simulink model "FMCW_Target_Emulator_RevA"  (R2021b)
settings: Solver=VariableStepAuto  StartTime=0.0  StopTime=stop_time  RelTol=1e-3
values from neighbouring files (symbols this model uses):
  simulator = Simulator_revB()    [compute_sensed_targets.m]    (also in compute_sensed_values.m)
undefined symbols (not defined in the file or in its folder): emulated_target
libraries: hdlsllib x2, simulink x1
settings Model: SimulationMode=accelerator  Creator=David  LastModifiedBy=David

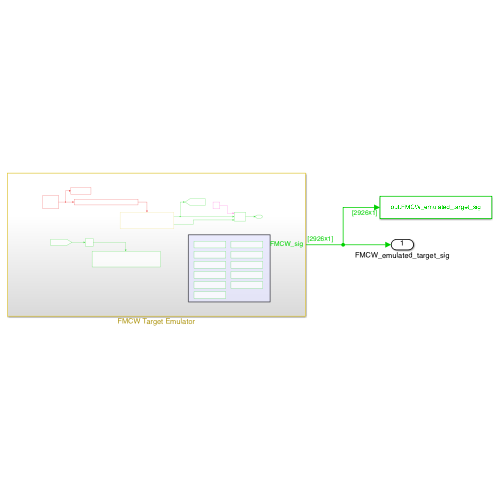
[thumbnail: Simulink's stored preview of the top-level diagram]
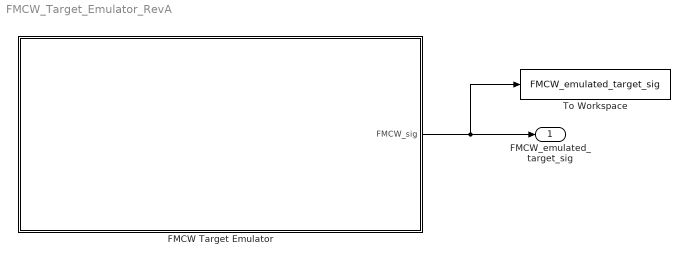
== system FMCW_Target_Emulator_RevA ==
  FMCW Target Emulator : Subsystem
  To Workspace : ToWorkspace  VariableName=FMCW_emulated_target_sig  SampleTime=-1
      settings: MaxDataPoints=2
  FMCW_emulated_target_sig : Outport
  wires:
  FMCW Target Emulator/1(FMCW_sig) -> FMCW_emulated_target_sig/1, To Workspace/1

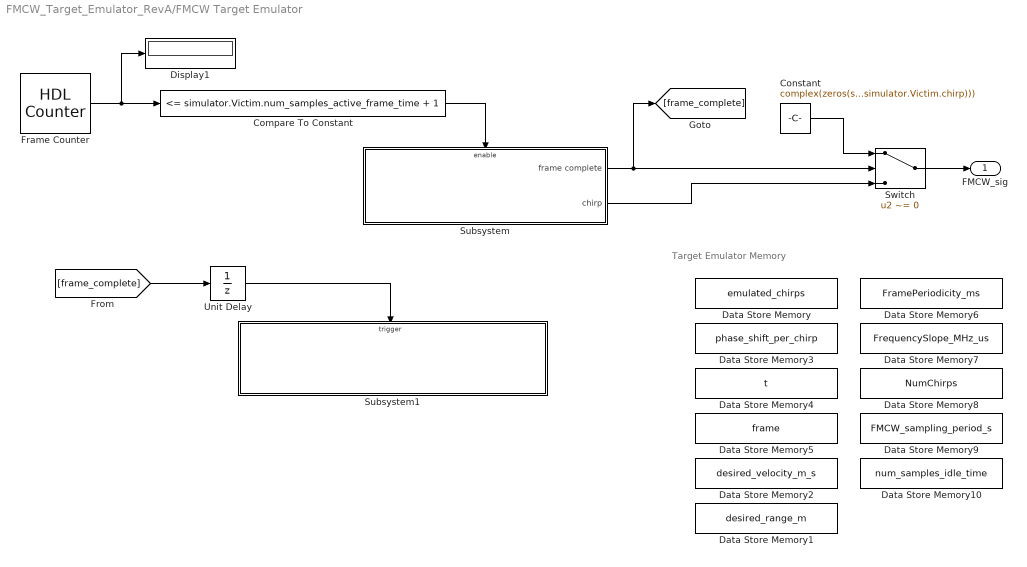
== system FMCW_Target_Emulator_RevA/FMCW Target Emulator ==
  note: Target Emulator Memory
  Compare To Constant : simulink/Logic and Bit Operations/Compare To Constant  relop=<=  const=simulator.Victim.num_samples_active_frame_time + 1  OutDataTypeStr=boolean
  Constant : Constant  Value=complex(zeros(size(simulator.Victim.chirp)))  VectorParams1D=off
  Data Store Memory : DataStoreMemory  DataStoreName=emulated_chirps  ReadBeforeWriteMsg=warning  WriteAfterWriteMsg=warning  WriteAfterReadMsg=warning  InitialValue=emulated_target.emulated_chirps  VectorParams1D=off  ShowAdditionalParam=off  OutDataTypeStr=double  Dimensions=size(emulated_target.emulated_chirps)
      settings: SignalType=complex
  Data Store Memory1 : DataStoreMemory  DataStoreName=desired_range_m  ReadBeforeWriteMsg=warning  WriteAfterWriteMsg=warning  WriteAfterReadMsg=warning  InitialValue=emulated_target.desired_range_m  ShowAdditionalParam=off  OutDataTypeStr=double
  Data Store Memory10 : DataStoreMemory  DataStoreName=num_samples_idle_time  ReadBeforeWriteMsg=warning  WriteAfterWriteMsg=warning  WriteAfterReadMsg=warning  InitialValue=emulated_target.Radar.num_samples_idle_time  ShowAdditionalParam=off  OutDataTypeStr=double
  Data Store Memory2 : DataStoreMemory  DataStoreName=desired_velocity_m_s  ReadBeforeWriteMsg=warning  WriteAfterWriteMsg=warning  WriteAfterReadMsg=warning  InitialValue=emulated_target.desired_velocity_m_s  ShowAdditionalParam=off  OutDataTypeStr=double
  Data Store Memory3 : DataStoreMemory  DataStoreName=phase_shift_per_chirp  ReadBeforeWriteMsg=warning  WriteAfterWriteMsg=warning  WriteAfterReadMsg=warning  InitialValue=emulated_target.phase_shift_per_chirp  ShowAdditionalParam=off  OutDataTypeStr=double
  Data Store Memory4 : DataStoreMemory  DataStoreName=t  ReadBeforeWriteMsg=warning  WriteAfterWriteMsg=warning  WriteAfterReadMsg=warning  InitialValue=emulated_target.t  ShowAdditionalParam=off  OutDataTypeStr=double  Dimensions=size(emulated_target.t)
  Data Store Memory5 : DataStoreMemory  DataStoreName=frame  ReadBeforeWriteMsg=warning  WriteAfterWriteMsg=warning  WriteAfterReadMsg=warning  InitialValue=1  ShowAdditionalParam=off  OutDataTypeStr=double
  Data Store Memory6 : DataStoreMemory  DataStoreName=FramePeriodicity_ms  ReadBeforeWriteMsg=warning  WriteAfterWriteMsg=warning  WriteAfterReadMsg=warning  InitialValue=emulated_target.Radar.FramePeriodicity_ms  ShowAdditionalParam=off  OutDataTypeStr=double
  Data Store Memory7 : DataStoreMemory  DataStoreName=FrequencySlope_MHz_us  ReadBeforeWriteMsg=warning  WriteAfterWriteMsg=warning  WriteAfterReadMsg=warning  InitialValue=emulated_target.Radar.FrequencySlope_MHz_us  ShowAdditionalParam=off  OutDataTypeStr=double
  Data Store Memory8 : DataStoreMemory  DataStoreName=NumChirps  ReadBeforeWriteMsg=warning  WriteAfterWriteMsg=warning  WriteAfterReadMsg=warning  InitialValue=emulated_target.Radar.NumChirps  ShowAdditionalParam=off  OutDataTypeStr=int32
  Data Store Memory9 : DataStoreMemory  DataStoreName=FMCW_sampling_period_s  ReadBeforeWriteMsg=warning  WriteAfterWriteMsg=warning  WriteAfterReadMsg=warning  InitialValue=emulated_target.Radar.FMCW_sampling_period_s  ShowAdditionalParam=off  OutDataTypeStr=double
  Display1 : Display
  Frame Counter : hdlsllib/Sources/HDL Counter  CountType=Count limited  CountInit=1  CountStep=1  CountMax=simulator.Victim.num_samples_per_frame  CountFromType=Initial value  CountFrom=1  CountResetPort=off  CountLoadPort=off  CountEnbPort=off  CountDirPort=off  CountHitOutputPort=off  CountDataType=Unsigned  CountWordLen=32  CountFracLen=0  CountSampTime=1/simulator.Victim.FMCW_sampling_rate_Hz
  Subsystem : Subsystem
  Subsystem1 : Subsystem
  Switch : Switch  Criteria=u2 ~= 0
  Unit Delay : UnitDelay  SampleTime=-1  HasFrameUpgradeWarning=on
  FMCW_sig : Outport
  wires:
  Switch/1 -> FMCW_sig/1
  Constant/1 -> Switch/1
  Subsystem/2(chirp) -> Switch/3
  Compare To Constant/1 -> Subsystem/Enable
  Frame Counter/1 -> Compare To Constant/1, Display1/1
  Subsystem/1(frame complete) -> [frame_complete], Switch/2
  [frame_complete] -> Unit Delay/1
  Unit Delay/1 -> Subsystem1/Trigger

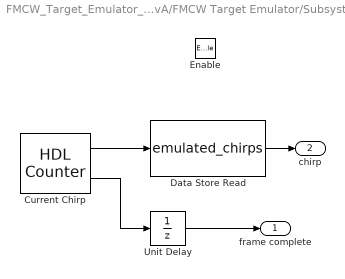
== system FMCW_Target_Emulator_RevA/FMCW Target Emulator/Subsystem ==
  Enable : EnablePort  StatesWhenEnabling=reset
  Current Chirp : hdlsllib/Sources/HDL Counter  CountType=Count limited  CountInit=1  CountStep=1  CountMax=simulator.Victim.NumChirps  CountFromType=Initial value  CountFrom=1  CountResetPort=off  CountLoadPort=off  CountEnbPort=off  CountDirPort=off  CountHitOutputPort=on  CountDataType=Signed  CountWordLen=32  CountFracLen=0  CountSampTime=simulator.Victim.ChirpCycleTime_us * 1e-6
  Data Store Read : DataStoreRead  DataStoreName=emulated_chirps  DataStoreElements=emulated_chirps  EnableIndexing=on  NumberOfDimensions=2  IndexOptions=Select all,Index vector (port)  Indices=1,1  OutputSizes=1,1
  Unit Delay : UnitDelay  SampleTime=-1  HasFrameUpgradeWarning=on
  frame complete : Outport
  chirp : Outport  Port=2  OutputWhenDisabled=reset  InitialOutput=complex(zeros(size(emulated_target.emulated_chirps(:,1))))
  wires:
  Current Chirp/1 -> Data Store Read/1
  Current Chirp/2 -> Unit Delay/1
  Data Store Read/1 -> chirp/1
  Unit Delay/1 -> frame complete/1

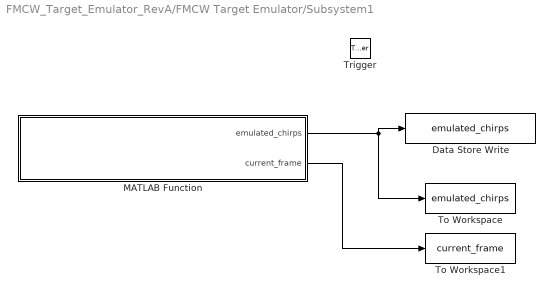
== system FMCW_Target_Emulator_RevA/FMCW Target Emulator/Subsystem1 ==
  Trigger : TriggerPort  VariantControl=(inherit)  PortDimensions=1
  Data Store Write : DataStoreWrite  DataStoreName=emulated_chirps  IndexOptions=Index vector (dialog)  Indices=1  OutputSizes=1
  MATLAB Function : MATLAB Function  TreatAsAtomicUnit=on
  To Workspace : ToWorkspace  VariableName=emulated_chirps  SampleTime=-1
      settings: MaxDataPoints=2
  To Workspace1 : ToWorkspace  VariableName=current_frame  SampleTime=-1
      settings: MaxDataPoints=2
  wires:
  MATLAB Function/1(emulated_chirps) -> Data Store Write/1, To Workspace/1
  MATLAB Function/2(current_frame) -> To Workspace1/1

== matlab function FMCW_Target_Emulator_RevA/FMCW Target Emulator/Subsystem1/MATLAB Function ==
  data: t data_store_memory; phase_shift_per_chirp data_store_memory; desired_range_m data_store_memory; desired_velocity_m_s data_store_memory; frame data_store_memory; FramePeriodicity_ms data_store_memory; FrequencySlope_MHz_us data_store_memory; NumChirps data_store_memory; FMCW_sampling_period_s data_store_memory; num_samples_idle_time data_store_memory; emulated_chirps_size parameter; emulated_chirps output; current_frame output
function [emulated_chirps,current_frame] = compute_next_emulated_chirps(emulated_chirps_size)
    
    global phase_shift_per_chirp
    global t

    global desired_range_m
    global desired_velocity_m_s

    global frame

    %the following variables provide necessary information on the radar to
    %implement
    global FramePeriodicity_ms
    global FrequencySlope_MHz_us
    global NumChirps
    global FMCW_sampling_period_s
    global num_samples_idle_time

    frame = frame + 1;
    current_frame = frame;
    emulated_chirps = complex(zeros(emulated_chirps_size));
    
    %time delay for current emulation range
    current_emulation_range = desired_range_m - ...
        desired_velocity_m_s * ...
        FramePeriodicity_ms * 1e-3 * ...
        (double(frame) - 1);
    time_delay = range2time(current_emulation_range,physconst('lightspeed'));
    num_samples_delay = time_delay / FMCW_sampling_period_s;
    
    for chirp = 1:int32(NumChirps)
        %compute the phase shift
        phase_shift = (double(chirp) - 1) * phase_shift_per_chirp;
    
        %compute the waveform
        waveform = cos(pi * FrequencySlope_MHz_us * 1e12 ...
            * t.^(2) + phase_shift) + ...
            1i * sin(pi * FrequencySlope_MHz_us ...
            * t.^(2) + phase_shift);
    
        %save it in the attacker_chirps array
        emulated_chirps(num_samples_idle_time + 1:end,chirp) = waveform.';
    
        if int32(num_samples_delay) > 0
            emulated_chirps(:,chirp) = ...
                [zeros(int32(num_samples_delay),1);...
                emulated_chirps(1: end - int32(num_samples_delay),chirp)];
        elseif num_samples_delay < 0
                emulated_chirps(:,chirp) = ...
                [emulated_chirps(int32(-1 * num_samples_delay) + 1: end,chirp);...
                zeros(int32(-1 * num_samples_delay),1)];
        end
    end
end
